simulink model "project_2"  (R2019a)
settings: Solver=VariableStepAuto  StartTime=0.0  StopTime=10.0  RelTol=1e-3
values from neighbouring files (symbols this model uses):
  A = 3    [project_2_run.m]
  F = 2    [project_2_run.m]    (also in project_3.m = 1; project_4_run.m = 1)
  Ti = .5    (= 0.5)    [project_2_run.m]
settings Model: Creator=Nikita  LastModifiedBy=Nikita

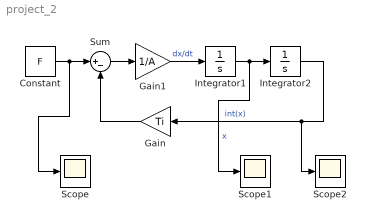
== system project_2 ==
  Constant : Constant  Value=F
  Gain : Gain  Gain=Ti
  Gain1 : Gain  Gain=1/A
  Integrator1 : Integrator
  Integrator2 : Integrator
  Scope : Scope
  Scope1 : Scope
  Scope2 : Scope
  Sum : Sum  Inputs=|+-
  wires:
  Gain1/1 -> Integrator1/1  "dx/dt"
  Integrator1/1 -> Scope1/1, Integrator2/1  "x"
  Integrator2/1 -> Scope2/1, Gain/1  "int(x)"
  Constant/1 -> Scope/1, Sum/1
  Gain/1 -> Sum/2
  Sum/1 -> Gain1/1
